simulink model "Modeliranje_i_upravljanje_letjelicom_starter_pack_plain"  (R2019b)
settings: Solver=VariableStepAuto  StartTime=0.0  StopTime=5  RelTol=1e-3
values from neighbouring files (symbols this model uses):
  k_p2 = 1.005572    [Modeliranje_i_upravljanje_letjelicom_starterpack.m]
  k_r2 = 1.001888    [Modeliranje_i_upravljanje_letjelicom_starterpack.m]
  k_y2 = 1.0    (= 1)    [Modeliranje_i_upravljanje_letjelicom_starterpack.m]
  k_z = 6.066    [Modeliranje_i_upravljanje_letjelicom_starterpack.m]
  wn_p2 = 10.672720    (= 10.67272)    [Modeliranje_i_upravljanje_letjelicom_starterpack.m]
  wn_r2 = 12.485386    [Modeliranje_i_upravljanje_letjelicom_starterpack.m]
  wn_y2 = 9.875759    [Modeliranje_i_upravljanje_letjelicom_starterpack.m]
  wn_z = 6.26    [Modeliranje_i_upravljanje_letjelicom_starterpack.m]
  zeta_p2 = 1.000000    (= 1)    [Modeliranje_i_upravljanje_letjelicom_starterpack.m]
  zeta_r2 = 1.000000    (= 1)    [Modeliranje_i_upravljanje_letjelicom_starterpack.m]
  zeta_y2 = 1.000000    (= 1)    [Modeliranje_i_upravljanje_letjelicom_starterpack.m]
settings Model: Creator=robert  LastModifiedBy=Filip

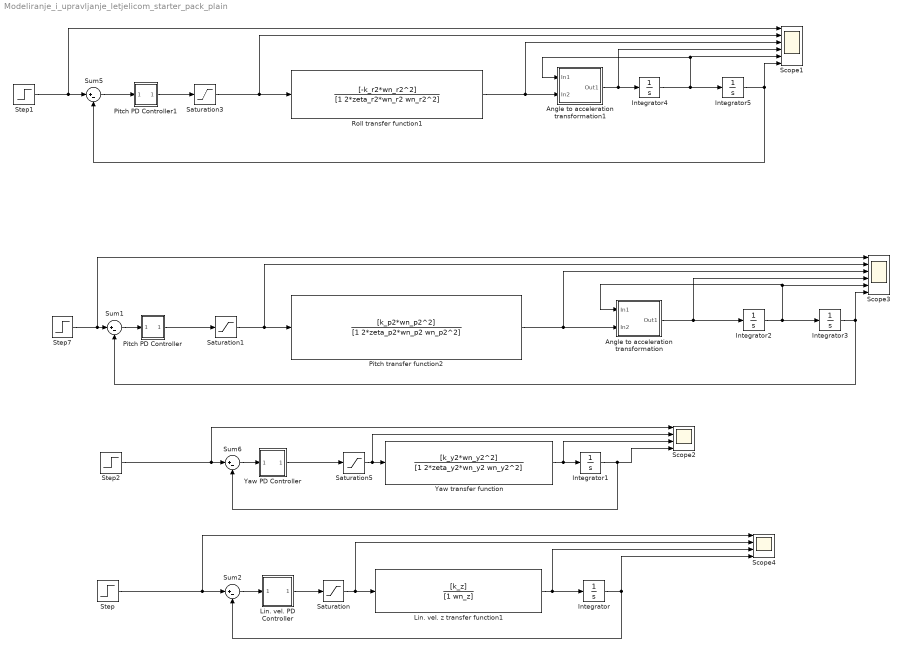
== system Modeliranje_i_upravljanje_letjelicom_starter_pack_plain ==
  Angle to acceleration transformation : Subsystem
  Angle to acceleration transformation1 : Subsystem
  Integrator{,1..5} (6 alike) : Integrator
  Lin. vel. PD Controller : Subsystem
  Lin. vel. z transfer function1 : TransferFcn  Numerator=[k_z]  Denominator=[1 wn_z]
  Pitch PD Controller : Subsystem
  Pitch PD Controller1 : Subsystem
  Pitch transfer function2 : TransferFcn  Numerator=[k_p2*wn_p2^2]  Denominator=[1 2*zeta_p2*wn_p2 wn_p2^2]
  Roll transfer function1 : TransferFcn  Numerator=[-k_r2*wn_r2^2]  Denominator=[1 2*zeta_r2*wn_r2 wn_r2^2]
  Saturation : Saturate  UpperLimit=3  LowerLimit=-3
  Saturation1 : Saturate  UpperLimit=30  LowerLimit=-30
  Saturation3 : Saturate  UpperLimit=30  LowerLimit=-30
  Saturation5 : Saturate  UpperLimit=80  LowerLimit=-80
  Scope1 : Scope  NumInputPorts=6
  Scope2 : Scope  NumInputPorts=4
  Scope3 : Scope  NumInputPorts=6
  Scope4 : Scope  NumInputPorts=4
  Step : Step  Time=0  After=2  SampleTime=0
  Step1 : Step  Time=0  After=0.5  SampleTime=0
  Step2 : Step  Time=0  After=45  SampleTime=0
  Step7 : Step  Time=0  After=5  SampleTime=0
  Sum{1..2,5..6} (4 alike) : Sum  Inputs=|+-
  Yaw PD Controller : Subsystem
  Yaw transfer function : TransferFcn  Numerator=[k_y2*wn_y2^2]  Denominator=[1 2*zeta_y2*wn_y2 wn_y2^2]
  wires:
  Lin. vel. z transfer function1/1 -> Scope4/3, Integrator/1
  Integrator/1 -> Sum2/2, Scope4/4
  Saturation/1 -> Scope4/2, Lin. vel. z transfer function1/1
  Yaw transfer function/1 -> Scope2/3, Integrator1/1
  Integrator3/1 -> Sum1/2, Scope3/6
  Pitch transfer function2/1 -> Scope3/3, Angle to acceleration transformation/2(In2)
  Saturation1/1 -> Scope3/2, Pitch transfer function2/1
  Integrator2/1 -> Angle to acceleration transformation/1(In1), Scope3/5, Integrator3/1
  Integrator1/1 -> Scope2/4, Sum6/2
  Step1/1 -> Scope1/1, Sum5/1
  Sum5/1 -> Pitch PD Controller1/1("  ")
  Saturation3/1 -> Scope1/2, Roll transfer function1/1
  Roll transfer function1/1 -> Scope1/3, Angle to acceleration transformation1/2(In2)
  Pitch PD Controller1/1(" ") -> Saturation3/1
  Saturation5/1 -> Scope2/2, Yaw transfer function/1
  Lin. vel. PD Controller/1(" ") -> Saturation/1
  Yaw PD Controller/1("  ") -> Saturation5/1
  Step2/1 -> Scope2/1, Sum6/1
  Sum6/1 -> Yaw PD Controller/1(" ")
  Angle to acceleration transformation/1(Out1) -> Scope3/4, Integrator2/1
  Pitch PD Controller/1(" ") -> Saturation1/1
  Step7/1 -> Scope3/1, Sum1/1
  Sum1/1 -> Pitch PD Controller/1("  ")
  Angle to acceleration transformation1/1(Out1) -> Scope1/4, Integrator4/1
  Integrator4/1 -> Scope1/5, Angle to acceleration transformation1/1(In1), Integrator5/1
  Integrator5/1 -> Scope1/6, Sum5/2
  Sum2/1 -> Lin. vel. PD Controller/1("  ")
  Step/1 -> Scope4/1, Sum2/1

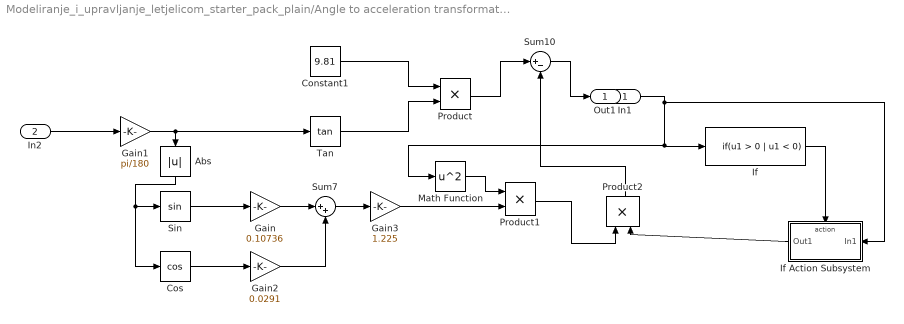
== system Modeliranje_i_upravljanje_letjelicom_starter_pack_plain/Angle to acceleration transformation ==
  In1 : Inport
  In2 : Inport  Port=2
  Abs : Abs
  Constant1 : Constant  Value=9.81
  Cos : Trigonometry  Operator=cos
  Gain : Gain  Gain=0.10736
  Gain1 : Gain  Gain=pi/180
  Gain2 : Gain  Gain=0.0291
  Gain3 : Gain  Gain=1.225
  If : If  IfExpression=u1 > 0 | u1 < 0  ShowElse=off
  If Action Subsystem : Subsystem  TreatAsAtomicUnit=on
  Math Function : Math  Operator=square  SignedPower=off  SaturateOnIntegerOverflow=on
  Product : Product
  Product1 : Product
  Product2 : Product
  Sin : Trigonometry
  Sum10 : Sum  Inputs=|+-
  Sum7 : Sum  Inputs=|++
  Tan : Trigonometry  Operator=tan
  Out1 : Outport
  wires:
  Constant1/1 -> Product/1
  Sum7/1 -> Gain3/1
  Gain3/1 -> Product1/2
  Product1/1 -> Product2/1
  Tan/1 -> Product/2
  Cos/1 -> Gain2/1
  Product/1 -> Sum10/1
  Gain/1 -> Sum7/1
  Sin/1 -> Gain/1
  Math Function/1 -> Product1/1
  Gain2/1 -> Sum7/2
  In2/1 -> Gain1/1
  Sum10/1 -> Out1/1
  In1/1 -> If Action Subsystem/1(In1), Math Function/1, If/1
  Gain1/1 -> Abs/1, Tan/1
  If Action Subsystem/1(Out1) -> Product2/2
  Product2/1 -> Sum10/2
  If/1 -> If Action Subsystem/Action
  Abs/1 -> Cos/1, Sin/1

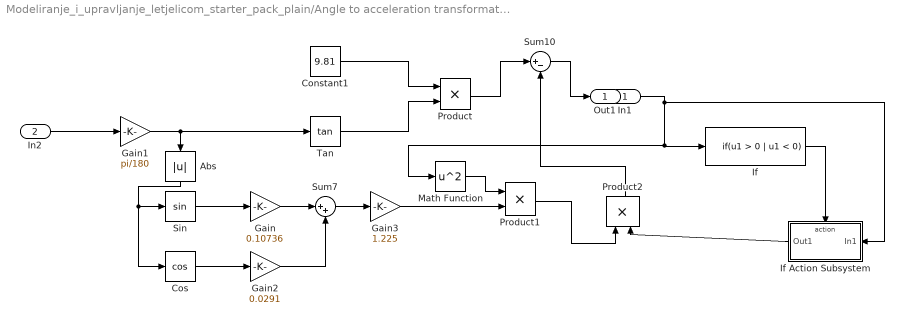
== system Modeliranje_i_upravljanje_letjelicom_starter_pack_plain/Angle to acceleration transformation1 ==
  In1 : Inport
  In2 : Inport  Port=2
  Abs : Abs
  Constant1 : Constant  Value=9.81
  Cos : Trigonometry  Operator=cos
  Gain : Gain  Gain=0.10736
  Gain1 : Gain  Gain=pi/180
  Gain2 : Gain  Gain=0.0291
  Gain3 : Gain  Gain=1.225
  If : If  IfExpression=u1 > 0 | u1 < 0  ShowElse=off
  If Action Subsystem : Subsystem  TreatAsAtomicUnit=on
  Math Function : Math  Operator=square  SignedPower=off  SaturateOnIntegerOverflow=on
  Product : Product
  Product1 : Product
  Product2 : Product
  Sin : Trigonometry
  Sum10 : Sum  Inputs=|+-
  Sum7 : Sum  Inputs=|++
  Tan : Trigonometry  Operator=tan
  Out1 : Outport
  wires:
  If/1 -> If Action Subsystem/Action
  Product2/1 -> Sum10/2
  If Action Subsystem/1(Out1) -> Product2/2
  Gain1/1 -> Abs/1, Tan/1
  In1/1 -> If/1, Math Function/1, If Action Subsystem/1(In1)
  Sum10/1 -> Out1/1
  In2/1 -> Gain1/1
  Gain2/1 -> Sum7/2
  Math Function/1 -> Product1/1
  Sin/1 -> Gain/1
  Gain/1 -> Sum7/1
  Product/1 -> Sum10/1
  Cos/1 -> Gain2/1
  Tan/1 -> Product/2
  Product1/1 -> Product2/1
  Gain3/1 -> Product1/2
  Sum7/1 -> Gain3/1
  Constant1/1 -> Product/1
  Abs/1 -> Cos/1, Sin/1

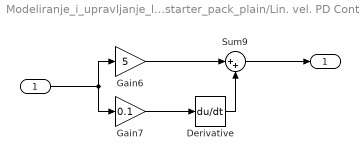
== system Modeliranje_i_upravljanje_letjelicom_starter_pack_plain/Lin. vel. PD Controller ==
  "  " : Inport
  Derivative : Derivative
  Gain6 : Gain  Gain=5
  Gain7 : Gain  Gain=0.1
  Sum9 : Sum  Inputs=|++
  " " : Outport
  wires:
  "  "/1 -> Gain7/1, Gain6/1
  Derivative/1 -> Sum9/2
  Gain6/1 -> Sum9/1
  Gain7/1 -> Derivative/1
  Sum9/1 -> " "/1

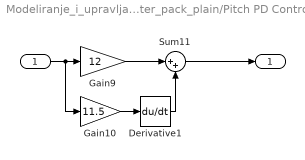
== system Modeliranje_i_upravljanje_letjelicom_starter_pack_plain/Pitch PD Controller ==
  "  " : Inport
  Derivative1 : Derivative
  Gain10 : Gain  Gain=11.5
  Gain9 : Gain  Gain=12
  Sum11 : Sum  Inputs=|++
  " " : Outport
  wires:
  Gain9/1 -> Sum11/1
  Gain10/1 -> Derivative1/1
  "  "/1 -> Gain10/1, Gain9/1
  Derivative1/1 -> Sum11/2
  Sum11/1 -> " "/1

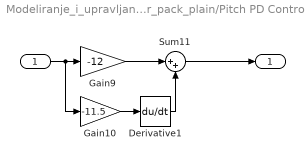
== system Modeliranje_i_upravljanje_letjelicom_starter_pack_plain/Pitch PD Controller1 ==
  "  " : Inport
  Derivative1 : Derivative
  Gain10 : Gain  Gain=-11.5
  Gain9 : Gain  Gain=-12
  Sum11 : Sum  Inputs=|++
  " " : Outport
  wires:
  Sum11/1 -> " "/1
  Derivative1/1 -> Sum11/2
  "  "/1 -> Gain9/1, Gain10/1
  Gain10/1 -> Derivative1/1
  Gain9/1 -> Sum11/1

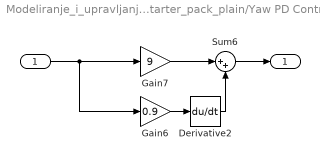
== system Modeliranje_i_upravljanje_letjelicom_starter_pack_plain/Yaw PD Controller ==
  " " : Inport
  Derivative2 : Derivative
  Gain6 : Gain  Gain=0.9
  Gain7 : Gain  Gain=9
  Sum6 : Sum  Inputs=|++
  "  " : Outport
  wires:
  Gain7/1 -> Sum6/1
  Gain6/1 -> Derivative2/1
  " "/1 -> Gain6/1, Gain7/1
  Derivative2/1 -> Sum6/2
  Sum6/1 -> "  "/1

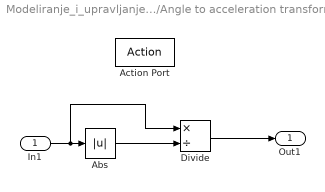
== system Modeliranje_i_upravljanje_letjelicom_starter_pack_plain/Angle to acceleration transformation/If Action Subsystem ==
  In1 : Inport
  Action Port : ActionPort  ActionPortLabel=if(u1 > 0 | u1 < 0)
  Abs : Abs
  Divide : Product  Inputs=*/
  Out1 : Outport
  wires:
  Abs/1 -> Divide/2
  In1/1 -> Divide/1, Abs/1
  Divide/1 -> Out1/1

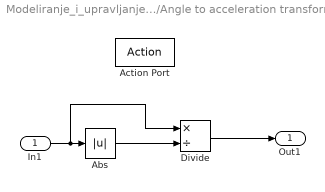
== system Modeliranje_i_upravljanje_letjelicom_starter_pack_plain/Angle to acceleration transformation1/If Action Subsystem ==
  In1 : Inport
  Action Port : ActionPort  ActionPortLabel=if(u1 > 0 | u1 < 0)
  Abs : Abs
  Divide : Product  Inputs=*/
  Out1 : Outport
  wires:
  Divide/1 -> Out1/1
  In1/1 -> Abs/1, Divide/1
  Abs/1 -> Divide/2
